simulink model "Earth_sim"  (R2024b)
settings: Solver=VariableStepAuto  StartTime=0.0  StopTime=15e4  FixedStep=0.5  MaxStep=max_step_size  RelTol=1e-6
values from neighbouring files (symbols this model uses):
  Earth_planet = Planet(mu,R,s,obliquity,deg2rad(9))    [Earth_setup.m]
  escape_data = escape(Earth_planet,launch_site,launch_data,transfer_data,orbit_plane_normal)    [Earth_setup.m]    (also in escape.m = struct("v_target", v_target,                       "time", t)
  launch_burn_time = 0.1    [Earth_setup.m]
  launch_data = struct("delta_t", delta_t,                       "v_target", v_target,                       "r_target", r_target,                       "ground2geo", ground2geo)    [launch2orbit.m]
  launch_site = Launch_Site("Kourou","Earth",deg2rad([5.264693257042033; -52.792193957435764]))    [Earth_setup.m]
  orbit_plane_normal = peri2geo*[0;0;1]    [Planet.m]    (also in launch2orbit.m)
  transfer_burn_time = 1    [Solar_system_setup.m]
libraries: simulink_extras x2
settings Model: Creator=cpero  LastModifiedBy=cpero
settings SolverCC: MaxConsecutiveMinStep=10  MinimalZcImpactIntegration=on  EnableFixedStepZeroCrossing=on
settings DebuggingCC: ReadBeforeWriteMsg=DisableAll  WriteAfterWriteMsg=DisableAll  WriteAfterReadMsg=DisableAll  MultiTaskDSMMsg=none
settings ModelReferenceCC: UpdateModelReferenceTargets=IfOutOfDate
settings SFSimCC: SFSimEcho=off

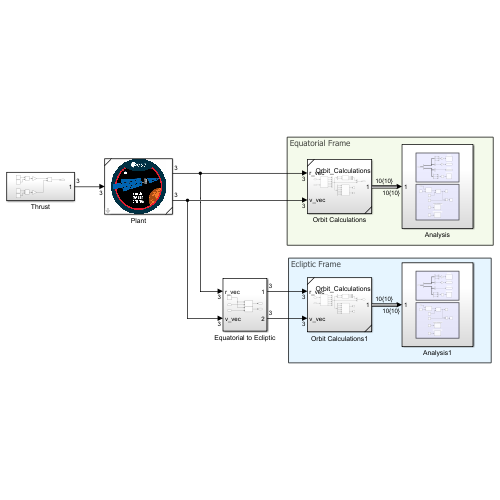
[thumbnail: Simulink's stored preview of the top-level diagram]
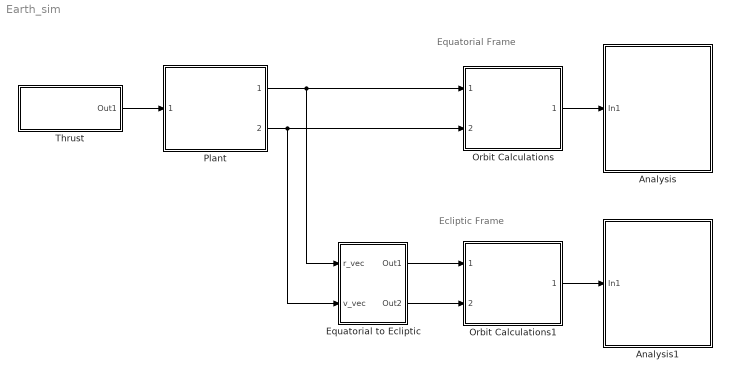
== system Earth_sim ==
  note: Equatorial Frame
  note: Ecliptic Frame
  Analysis : Subsystem
  Analysis1 : Subsystem
  Equatorial to Ecliptic : Subsystem
  Orbit Calculations : Subsystem  ReferencedSubsystem=Orbit_Calculations
  Orbit Calculations1 : Subsystem  ReferencedSubsystem=Orbit_Calculations
  Plant : Subsystem  ReferencedSubsystem=Plant  initial_data=launch_initial  maneuver_time=launch_data.delta_t  mu=Earth_planet.mu
  Thrust : Subsystem
  wires:
  Orbit Calculations/1 -> Analysis/1(In1)
  Plant/1 -> Orbit Calculations/1, Equatorial to Ecliptic/1(r_vec)
  Plant/2 -> Orbit Calculations/2, Equatorial to Ecliptic/2(v_vec)
  Orbit Calculations1/1 -> Analysis1/1(In1)
  Equatorial to Ecliptic/1(Out1) -> Orbit Calculations1/1
  Equatorial to Ecliptic/2(Out2) -> Orbit Calculations1/2
  Thrust/1(Out1) -> Plant/1

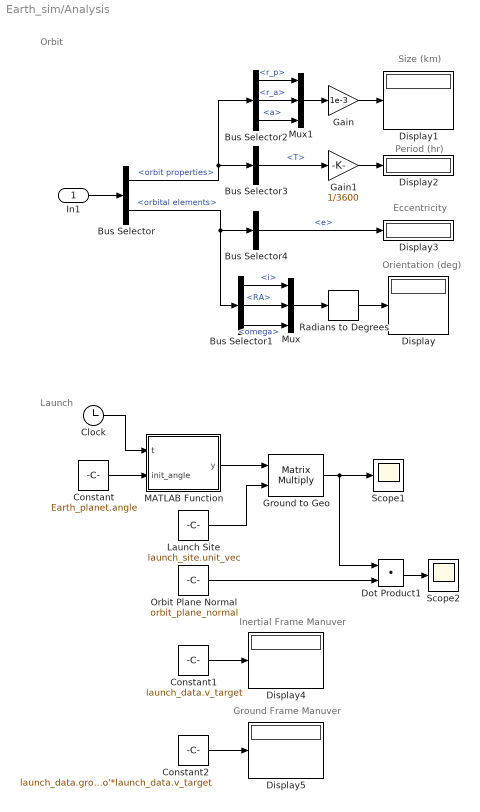
== system Earth_sim/Analysis ==
  note: Launch
  note: Orbit
  note: Period (hr)
  note: Orientation (deg)
  note: Size (km)
  note: Eccentricity
  note: Ground Frame Manuver
  note: Inertial Frame Manuver
  In1 : Inport
  Bus Selector : BusSelector  OutputSignals=orbit properties,orbital elements
  Bus Selector1 : BusSelector  OutputSignals=i,RA,omega
  Bus Selector2 : BusSelector  OutputSignals=r_p,r_a,a
  Bus Selector3 : BusSelector  OutputSignals=T
  Bus Selector4 : BusSelector  OutputSignals=e
  Clock : Clock
  Constant : Constant  Value=Earth_planet.angle
  Constant1 : Constant  Value=launch_data.v_target
  Constant2 : Constant  Value=launch_data.ground2geo'*launch_data.v_target
  Display{,1..5} (6 alike) : Display
  Dot Product1 : DotProduct  OutDataTypeStr=Inherit: Inherit via internal rule
  Gain : Gain  Gain=1e-3
  Gain1 : Gain  Gain=1/3600
  Ground to Geo : Product  Multiplication=Matrix(*)
  Launch Site : Constant  Value=launch_site.unit_vec
  MATLAB Function : MATLAB Function  TreatAsAtomicUnit=on
  Mux : Mux  Inputs=3
  Mux1 : Mux  Inputs=3
  Orbit Plane Normal : Constant  Value=orbit_plane_normal
  Radians to Degrees : simulink_extras/Transformations/Radians to Degrees
  Scope1 : Scope
  Scope2 : Scope
  wires:
  In1/1 -> Bus Selector/1
  Bus Selector/1 -> Bus Selector3/1, Bus Selector2/1  "<orbit properties>"
  Mux/1 -> Radians to Degrees/1
  Bus Selector/2 -> Bus Selector1/1, Bus Selector4/1  "<orbital elements>"
  Bus Selector1/1 -> Mux/1  "<i>"
  Bus Selector1/2 -> Mux/2  "<RA>"
  Radians to Degrees/1 -> Display/1
  Bus Selector1/3 -> Mux/3  "<omega>"
  Bus Selector2/1 -> Mux1/1  "<r_p>"
  Bus Selector2/2 -> Mux1/2  "<r_a>"
  Bus Selector2/3 -> Mux1/3  "<a>"
  Mux1/1 -> Gain/1
  Gain/1 -> Display1/1
  Bus Selector3/1 -> Gain1/1  "<T>"
  Gain1/1 -> Display2/1
  Bus Selector4/1 -> Display3/1  "<e>"
  Dot Product1/1 -> Scope2/1
  Orbit Plane Normal/1 -> Dot Product1/2
  Ground to Geo/1 -> Scope1/1, Dot Product1/1
  Clock/1 -> MATLAB Function/1(t)
  MATLAB Function/1(y) -> Ground to Geo/1
  Launch Site/1 -> Ground to Geo/2
  Constant2/1 -> Display5/1
  Constant1/1 -> Display4/1
  Constant/1 -> MATLAB Function/2(init_angle)

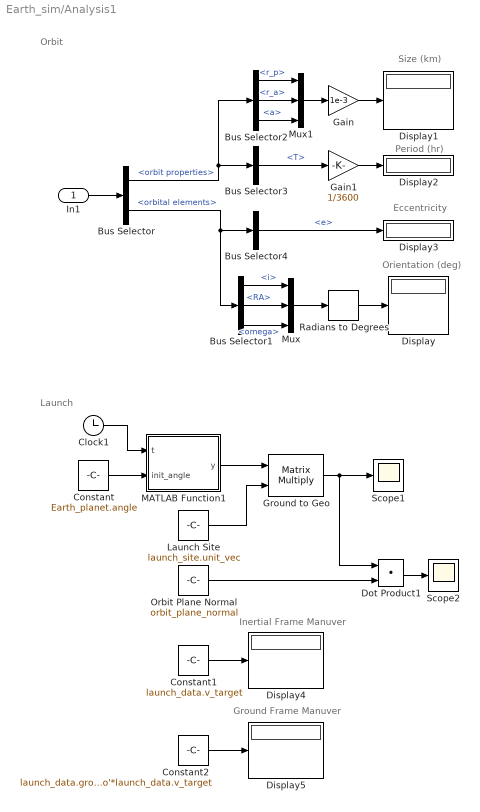
== system Earth_sim/Analysis1 ==
  note: Launch
  note: Orbit
  note: Period (hr)
  note: Orientation (deg)
  note: Size (km)
  note: Eccentricity
  note: Ground Frame Manuver
  note: Inertial Frame Manuver
  In1 : Inport
  Bus Selector : BusSelector  OutputSignals=orbit properties,orbital elements
  Bus Selector1 : BusSelector  OutputSignals=i,RA,omega
  Bus Selector2 : BusSelector  OutputSignals=r_p,r_a,a
  Bus Selector3 : BusSelector  OutputSignals=T
  Bus Selector4 : BusSelector  OutputSignals=e
  Clock1 : Clock
  Constant : Constant  Value=Earth_planet.angle
  Constant1 : Constant  Value=launch_data.v_target
  Constant2 : Constant  Value=launch_data.ground2geo'*launch_data.v_target
  Display{,1..5} (6 alike) : Display
  Dot Product1 : DotProduct  OutDataTypeStr=Inherit: Inherit via internal rule
  Gain : Gain  Gain=1e-3
  Gain1 : Gain  Gain=1/3600
  Ground to Geo : Product  Multiplication=Matrix(*)
  Launch Site : Constant  Value=launch_site.unit_vec
  MATLAB Function1 : MATLAB Function  TreatAsAtomicUnit=on
  Mux : Mux  Inputs=3
  Mux1 : Mux  Inputs=3
  Orbit Plane Normal : Constant  Value=orbit_plane_normal
  Radians to Degrees : simulink_extras/Transformations/Radians to Degrees
  Scope1 : Scope
  Scope2 : Scope
  wires:
  In1/1 -> Bus Selector/1
  Bus Selector/1 -> Bus Selector3/1, Bus Selector2/1  "<orbit properties>"
  Mux/1 -> Radians to Degrees/1
  Bus Selector/2 -> Bus Selector1/1, Bus Selector4/1  "<orbital elements>"
  Bus Selector1/1 -> Mux/1  "<i>"
  Bus Selector1/2 -> Mux/2  "<RA>"
  Radians to Degrees/1 -> Display/1
  Bus Selector1/3 -> Mux/3  "<omega>"
  Bus Selector2/1 -> Mux1/1  "<r_p>"
  Bus Selector2/2 -> Mux1/2  "<r_a>"
  Bus Selector2/3 -> Mux1/3  "<a>"
  Mux1/1 -> Gain/1
  Gain/1 -> Display1/1
  Bus Selector3/1 -> Gain1/1  "<T>"
  Gain1/1 -> Display2/1
  Bus Selector4/1 -> Display3/1  "<e>"
  Dot Product1/1 -> Scope2/1
  Orbit Plane Normal/1 -> Dot Product1/2
  Ground to Geo/1 -> Scope1/1, Dot Product1/1
  MATLAB Function1/1(y) -> Ground to Geo/1
  Launch Site/1 -> Ground to Geo/2
  Constant2/1 -> Display5/1
  Constant1/1 -> Display4/1
  Constant/1 -> MATLAB Function1/2(init_angle)
  Clock1/1 -> MATLAB Function1/1(t)

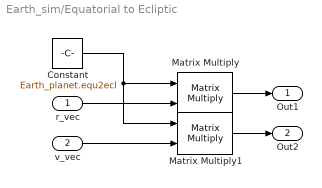
== system Earth_sim/Equatorial to Ecliptic ==
  r_vec : Inport
  v_vec : Inport  Port=2
  Constant : Constant  Value=Earth_planet.equ2ecl
  Matrix Multiply : Product  Multiplication=Matrix(*)
  Matrix Multiply1 : Product  Multiplication=Matrix(*)
  Out1 : Outport
  Out2 : Outport  Port=2
  wires:
  Constant/1 -> Matrix Multiply1/1, Matrix Multiply/1
  Matrix Multiply1/1 -> Out2/1
  Matrix Multiply/1 -> Out1/1
  r_vec/1 -> Matrix Multiply/2
  v_vec/1 -> Matrix Multiply1/2

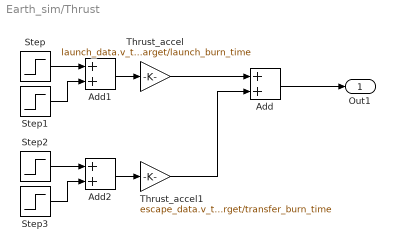
== system Earth_sim/Thrust ==
  Add : Sum
  Add1 : Sum
  Add2 : Sum
  Step : Step  Time=launch_data.delta_t  SampleTime=0
  Step1 : Step  Time=launch_data.delta_t + launch_burn_time  After=-1  SampleTime=0
  Step2 : Step  Time=launch_data.delta_t + escape_data.time  SampleTime=0
  Step3 : Step  Time=launch_data.delta_t + escape_data.time + transfer_burn_time  After=-1  SampleTime=0
  Thrust_accel : Gain  Gain=launch_data.v_target/launch_burn_time
  Thrust_accel1 : Gain  Gain=escape_data.v_target/transfer_burn_time
  Out1 : Outport
  wires:
  Add1/1 -> Thrust_accel/1
  Step2/1 -> Add2/1
  Step1/1 -> Add1/2
  Add2/1 -> Thrust_accel1/1
  Step3/1 -> Add2/2
  Step/1 -> Add1/1
  Thrust_accel/1 -> Add/1
  Thrust_accel1/1 -> Add/2
  Add/1 -> Out1/1

== matlab function Earth_sim/Analysis/MATLAB Function ==
  data: y output; t input; omega parameter; init_angle input
function y = fcn(t, omega, init_angle)

y = [cos(omega*t + init_angle), -sin(omega*t + init_angle), 0;
     sin(omega*t + init_angle), cos(omega*t + init_angle), 0;
     0, 0, 1];

== matlab function Earth_sim/Analysis1/MATLAB Function1 ==
  data: y output; t input; omega parameter; init_angle input
function y = fcn(t, omega, init_angle)

y = [cos(omega*t + init_angle), -sin(omega*t + init_angle), 0;
     sin(omega*t + init_angle), cos(omega*t + init_angle), 0;
     0, 0, 1];
